simulink model "PAM_SIM"  (R2024a)
settings: Solver=VariableStepAuto  StartTime=0.0  StopTime=1.0  RelTol=1e-3
libraries: dspfdesign x1
settings Model: Creator=adity  LastModifiedBy=adity

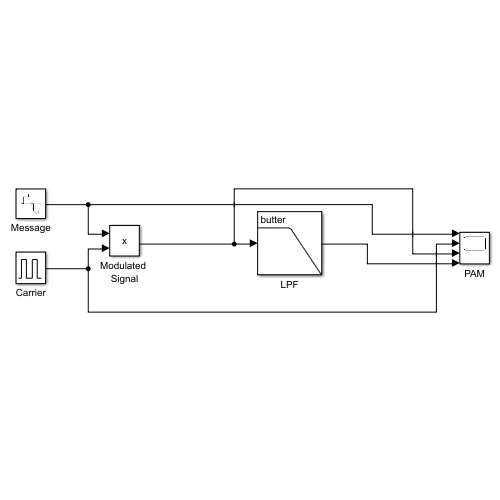
[thumbnail: Simulink's stored preview of the top-level diagram]
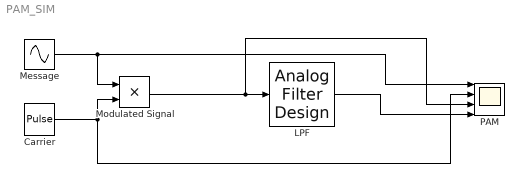
== system PAM_SIM ==
  Carrier : DiscretePulseGenerator  PulseType=Time based  Period=0.02  PulseWidth=50
  LPF : dspfdesign/Analog Filter Design  method=Butterworth  filttype=Lowpass  N=8  Wlo=30  Whi=80  Rp=2  Rs=40
  Message : Sin  Frequency=2*pi*1  SampleTime=1/1000
  Modulated Signal : Product
  PAM : Scope  NumInputPorts=4
  wires:
  Message/1 -> PAM/1, Modulated Signal/1
  Carrier/1 -> PAM/2, Modulated Signal/2
  Modulated Signal/1 -> PAM/3, LPF/1
  LPF/1 -> PAM/4
